simulink model "Signal_Processing"  (R2023b)
settings: Solver=FixedStepAuto  StartTime=0.0  StopTime=1  FixedStep=1e-4  RelTol=1e-3
libraries: simulink x2, spsRMSLib x2, spspowerguiLib x1
settings Model: Creator=Moisa Versatu  LastModifiedBy=Moisa Versatu

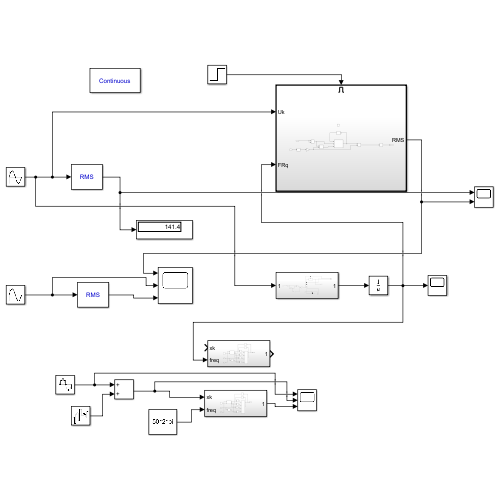
[thumbnail: Simulink's stored preview of the top-level diagram]
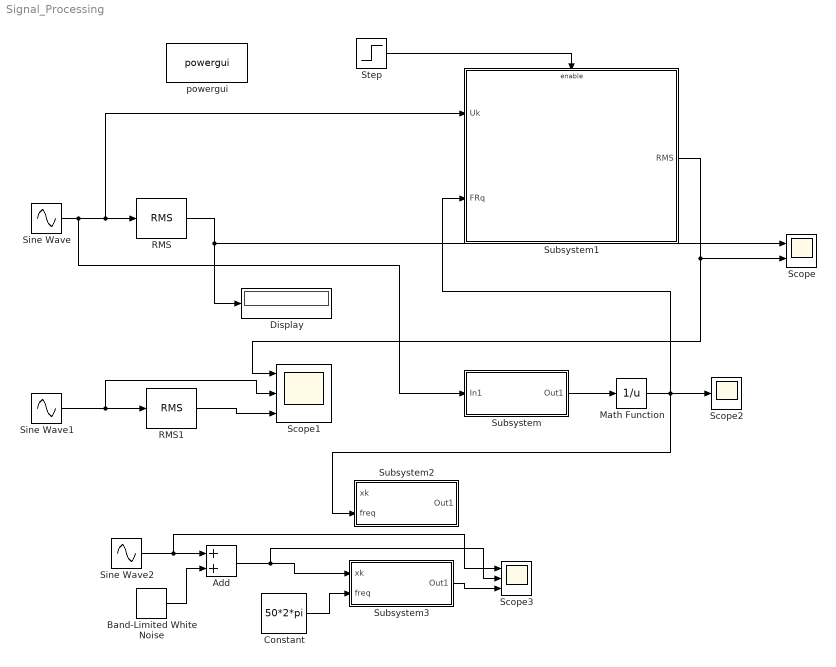
== system Signal_Processing ==
  Add : Sum
  Band-Limited White Noise : simulink/Sources/Band-Limited White Noise  Cov=[0.01]  Ts=1e-4  seed=[23341]
  Constant : Constant  Value=50*2*pi
  Display : Display
  Math Function : Math  Operator=reciprocal  SignedPower=on  RndMeth=Zero
  RMS : spsRMSLib/RMS  TrueRMS=on  Freq=50  RMSInit=0  Ts=0
  RMS1 : spsRMSLib/RMS  TrueRMS=on  Freq=50  RMSInit=0  Ts=0
  Scope : Scope  NumInputPorts=2
  Scope1 : Scope  NumInputPorts=3
  Scope2 : Scope
  Scope3 : Scope  NumInputPorts=3
  Sine Wave : Sin  Amplitude=200  Frequency=2*pi*50  SampleTime=0
  Sine Wave1 : Sin  Frequency=2*pi*50  SampleTime=0
  Sine Wave2 : Sin  Amplitude=200  Frequency=2*pi*50  SampleTime=1e-4
  Step : Step  Time=0.5  SampleTime=0
  Subsystem : Subsystem
  Subsystem1 : Subsystem
  Subsystem2 : Subsystem
  Subsystem3 : Subsystem
  powergui : spspowerguiLib/powergui  Priority=1  SimulationMode=Continuous  SampleTime=50e-6  frequency=60  Iterations=50  frequencyindice=60  Pbase=100e6  ErrMax=1e-4  UnitsV=kV  UnitsW=MW  buscounter=0  FunctionMessages=off  echomessages=off  EnableUseOfTLC=off  CurrentSourceSwitches=off  DisableSnubberDevices=off  DisableRonSwitches=off  DisableVfSwitches=off  DisplayEquations=off  AutomaticDiscreteSolvers=off  SolverType=Tustin/Backward Euler (TBE)  Interpol=off  ExternalGateDelay=off  methode=off  Ts=100  x0status=blocks  SPID=on  SwTol=0  HookPort=off  NonlinearTolerance=1e-4  nMaxIteration=100  ContinueOnMaxIteration=off  RestoreLinks=warning  ResistiveCurrentMeasurement=off  Frange=[0:2:500]  Ylog=off  Xlog=on  ShowGrid=off  save=off  variable=ZData  structure=0  ZoomFFT=off  StartTime=0.0  cycles=1  DisplayStyle=1  fundamental=60  FreqAxis=off  MaxFrequency=1000  frequencyindicesteady=1  RmsSteady=1  display=off
  wires:
  Sine Wave/1 -> Subsystem/1(In1), Subsystem1/1(Uk), RMS/1
  RMS/1 -> Display/1, Scope/1
  Sine Wave1/1 -> Scope1/2, RMS1/1
  RMS1/1 -> Scope1/3
  Subsystem1/1(RMS) -> Scope/2, Scope1/1
  Subsystem/1(Out1) -> Math Function/1
  Math Function/1 -> Subsystem2/2(freq), Scope2/1, Subsystem1/2(FRq)
  Step/1 -> Subsystem1/Enable
  Constant/1 -> Subsystem3/2(freq)
  Sine Wave2/1 -> Scope3/1, Add/1
  Add/1 -> Scope3/2, Subsystem3/1(xk)
  Band-Limited White Noise/1 -> Add/2
  Subsystem3/1(Out1) -> Scope3/3

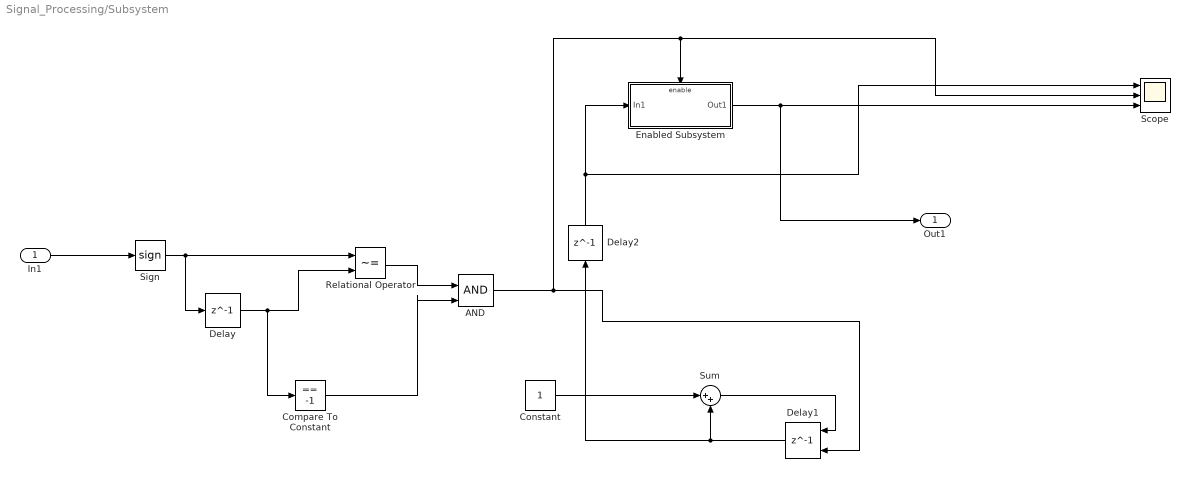
== system Signal_Processing/Subsystem ==
  In1 : Inport
  AND : Logic  IconShape=distinctive  AllPortsSameDT=off  OutDataTypeStr=boolean
  Compare To Constant : simulink/Logic and Bit Operations/Compare To Constant  relop===  const=-1  OutDataTypeStr=boolean
  Constant : Constant
  Delay : Delay  DelayLength=1
  Delay1 : Delay  DelayLength=1  ExternalReset=Rising
      settings: InputPortMap=u0,r5
  Delay2 : Delay  DelayLength=1
  Enabled Subsystem : Subsystem  TreatAsAtomicUnit=on
  Relational Operator : RelationalOperator  Operator=~=  OutDataTypeStr=boolean  RndMeth=Simplest  InputSameDT=off
  Scope : Scope  NumInputPorts=3
  Sign : Signum
  Sum : Sum  Inputs=|++
  Out1 : Outport
  wires:
  In1/1 -> Sign/1
  Sign/1 -> Relational Operator/1, Delay/1
  Delay/1 -> Compare To Constant/1, Relational Operator/2
  Relational Operator/1 -> AND/1
  Constant/1 -> Sum/1
  Delay1/1 -> Delay2/1, Sum/2
  Sum/1 -> Delay1/1
  Compare To Constant/1 -> AND/2
  AND/1 -> Delay1/2, Enabled Subsystem/Enable, Scope/2
  Enabled Subsystem/1(Out1) -> Scope/3, Out1/1
  Delay2/1 -> Scope/1, Enabled Subsystem/1(In1)

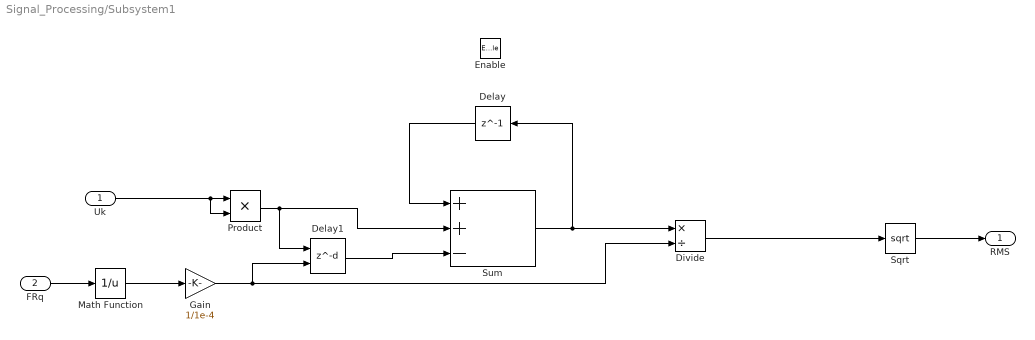
== system Signal_Processing/Subsystem1 ==
  Uk : Inport
  FRq : Inport  Port=2
  Enable : EnablePort
  Delay : Delay  DelayLength=1  InitialCondition=0
  Delay1 : Delay  DelayLengthSource=Input port  DelayLength=200  DelayLengthUpperLimit=500  InitialCondition=0
      settings: InputPortMap=u0,p1
  Divide : Product  Inputs=*/
  Gain : Gain  Gain=1/1e-4
  Math Function : Math  Operator=reciprocal  SignedPower=on  RndMeth=Zero
  Product : Product
  Sqrt : Sqrt
  Sum : Sum  Inputs=++-
  RMS : Outport
  wires:
  FRq/1 -> Math Function/1
  Sqrt/1 -> RMS/1
  Divide/1 -> Sqrt/1
  Uk/1 -> Product/1, Product/2
  Sum/1 -> Delay/1, Divide/1
  Delay/1 -> Sum/1
  Product/1 -> Sum/2, Delay1/1
  Delay1/1 -> Sum/3
  Math Function/1 -> Gain/1
  Gain/1 -> Delay1/2, Divide/2

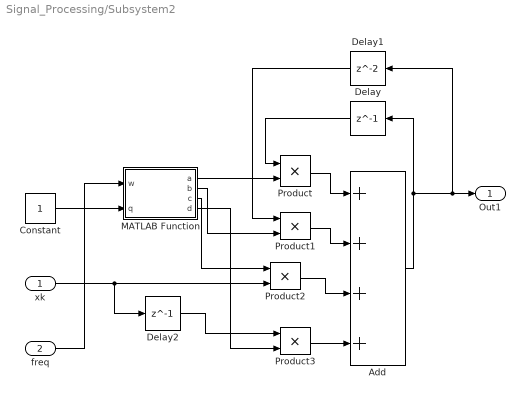
== system Signal_Processing/Subsystem2 ==
  xk : Inport
  freq : Inport  Port=2
  Add : Sum  Inputs=++++
  Constant : Constant
  Delay : Delay  DelayLength=1
  Delay1 : Delay
  Delay2 : Delay  DelayLength=1
  MATLAB Function : MATLAB Function  TreatAsAtomicUnit=on
  Product{,1..3} (4 alike) : Product
  Out1 : Outport
  wires:
  xk/1 -> Delay2/1, Product2/2
  MATLAB Function/4(d) -> Product3/2
  MATLAB Function/1(a) -> Product/2
  Product/1 -> Add/1
  Delay/1 -> Product/1
  Add/1 -> Delay1/1, Out1/1, Delay/1
  MATLAB Function/2(b) -> Product1/2
  Delay1/1 -> Product1/1
  Product1/1 -> Add/2
  MATLAB Function/3(c) -> Product2/1
  Product2/1 -> Add/3
  Delay2/1 -> Product3/1
  Product3/1 -> Add/4
  freq/1 -> MATLAB Function/1(w)
  Constant/1 -> MATLAB Function/2(q)

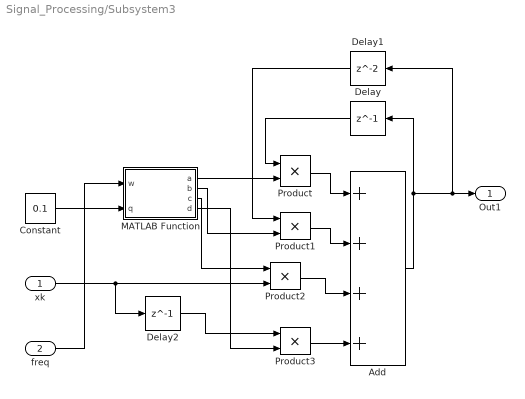
== system Signal_Processing/Subsystem3 ==
  xk : Inport
  freq : Inport  Port=2
  Add : Sum  Inputs=++++
  Constant : Constant  Value=0.1
  Delay : Delay  DelayLength=1
  Delay1 : Delay
  Delay2 : Delay  DelayLength=1
  MATLAB Function : MATLAB Function  TreatAsAtomicUnit=on
  Product{,1..3} (4 alike) : Product
  Out1 : Outport
  wires:
  Constant/1 -> MATLAB Function/2(q)
  freq/1 -> MATLAB Function/1(w)
  Product3/1 -> Add/4
  Product2/1 -> Add/3
  MATLAB Function/3(c) -> Product2/1
  Product1/1 -> Add/2
  Delay1/1 -> Product1/1
  MATLAB Function/2(b) -> Product1/2
  Add/1 -> Delay/1, Out1/1, Delay1/1
  Delay/1 -> Product/1
  Product/1 -> Add/1
  MATLAB Function/1(a) -> Product/2
  MATLAB Function/4(d) -> Product3/2
  xk/1 -> Delay2/1, Product2/2
  Delay2/1 -> Product3/1

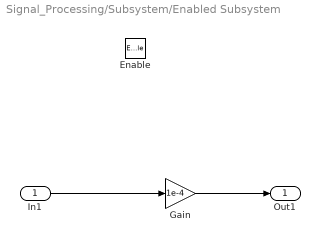
== system Signal_Processing/Subsystem/Enabled Subsystem ==
  In1 : Inport
  Enable : EnablePort
  Gain : Gain  Gain=1e-4
  Out1 : Outport
  wires:
  In1/1 -> Gain/1
  Gain/1 -> Out1/1

== matlab function Signal_Processing/Subsystem3/MATLAB Function ==
  data: w input; a output; q input; b output; c output; d output
function [a,b,c,d] = fcn(w,q)
a = (200000000*q + 10000*w)/(q*w^2 + 10000*w + 100000000*q);
b =-(100000000*q)/(q*w^2 + 10000*w + 100000000*q);
c =(10000*w)/(q*w^2 + 10000*w + 100000000*q);
d =-(10000*w)/(q*w^2 + 10000*w + 100000000*q);
end

== matlab function Signal_Processing/Subsystem2/MATLAB Function ==
  data: w input; a output; q input; b output; c output; d output
function [a,b,c,d] = fcn(w,q)
a = (200000000*q + 10000*w)/(q*w^2 + 10000*w + 100000000*q);
b =-(100000000*q)/(q*w^2 + 10000*w + 100000000*q);
c =(10000*w)/(q*w^2 + 10000*w + 100000000*q);
d =-(10000*w)/(q*w^2 + 10000*w + 100000000*q);
end
